simulink library "HEMERO"  (Simulink 3.00)
values from neighbouring files (symbols this model uses):
  K1 = 0.5    [ejh64.m]    (also in ejh65.m)
  K2 = 0.8    [ejh64.m]    (also in ejh65.m)
  x_camino = 0:0.01:10    [ejh64.m]    (also in ejh65.m)
  y_camino = x_camino.^2    [ejh64.m]    (also in ejh65.m)
undefined symbols (not defined in the file or in its folder): magnitude, nonlinear
libraries: simulink_extras x12, HEMERO x9, simulink3 x6, dspstat x4
(part 8 of 9)

== system HEMERO/Robots móviles/Control de robots móviles/Métodos basados en Teoría de Control/Seguimiento de trayectorias/Ejemplos/Ejemplo H.6.6/Seguimiento de trayectorias (Control lineal)/Control lineal/Cálculo de u1 ==
  e1 : Inport  Port=1  PortWidth=-1  SampleTime=-1  DataType=auto
      settings: SignalType=auto
  Gain : Gain  Gain=-K1  SaturateOnIntegerOverflow=on
  u1 : Outport  Port=1
  wires:
  e1/1 -> Gain/1
  Gain/1 -> u1/1

== system HEMERO/Robots móviles/Control de robots móviles/Métodos basados en Teoría de Control/Seguimiento de trayectorias/Ejemplos/Ejemplo H.6.6/Seguimiento de trayectorias (Control lineal)/Control lineal/Cálculo de u2  ==
  e2 : Inport  Port=1  PortWidth=-1  SampleTime=-1  DataType=auto
      settings: SignalType=auto
  e3 : Inport  Port=2  PortWidth=-1  SampleTime=-1  DataType=auto
      settings: SignalType=auto
  v_r : Inport  Port=3  PortWidth=-1  SampleTime=-1  DataType=auto
      settings: SignalType=auto
  Gain1 : Gain  Gain=-K2  SaturateOnIntegerOverflow=on
  Gain3 : Gain  Gain=-K3  SaturateOnIntegerOverflow=on
  Product1 : Product  Inputs=2  SaturateOnIntegerOverflow=on
  Sign : Signum
  Sum : Sum  Inputs=++  SaturateOnIntegerOverflow=on
  u2 : Outport  Port=1
  wires:
  Gain1/1 -> Product1/1
  Product1/1 -> Sum/1
  Sum/1 -> u2/1
  e3/1 -> Gain3/1
  Gain3/1 -> Sum/2
  e2/1 -> Gain1/1
  v_r/1 -> Sign/1
  Sign/1 -> Product1/2

== system HEMERO/Robots móviles/Control de robots móviles/Métodos basados en Teoría de Control/Seguimiento de trayectorias/Ejemplos/Ejemplo H.6.7/Seguimiento de trayectorias (Control lineal con escalado de velocidad)/Cambio de variable/Cálculo de e1 ==
  x_r : Inport  Port=1  PortWidth=-1  SampleTime=-1  DataType=auto
      settings: SignalType=auto
  x : Inport  Port=2  PortWidth=-1  SampleTime=-1  DataType=auto
      settings: SignalType=auto
  y_r : Inport  Port=3  PortWidth=-1  SampleTime=-1  DataType=auto
      settings: SignalType=auto
  y : Inport  Port=4  PortWidth=-1  SampleTime=-1  DataType=auto
      settings: SignalType=auto
  phi : Inport  Port=5  PortWidth=-1  SampleTime=-1  DataType=auto
      settings: SignalType=auto
  Product : Product  Inputs=2  SaturateOnIntegerOverflow=on
  Product1 : Product  Inputs=2  SaturateOnIntegerOverflow=on
  Sum : Sum  Inputs=-+  SaturateOnIntegerOverflow=on
  Sum1 : Sum  Inputs=+-  SaturateOnIntegerOverflow=on
  Sum2 : Sum  Inputs=++  SaturateOnIntegerOverflow=on
  Trigonometric Function : Trigonometry  Operator=sin  OutputSignalType=auto
  Trigonometric Function1 : Trigonometry  Operator=cos  OutputSignalType=auto
  e1 : Outport  Port=1
  wires:
  x_r/1 -> Sum/1
  x/1 -> Sum/2
  y_r/1 -> Sum1/1
  y/1 -> Sum1/2
  phi/1 -> Trigonometric Function/1, Trigonometric Function1/1
  Sum/1 -> Product/1
  Trigonometric Function/1 -> Product/2
  Sum1/1 -> Product1/1
  Trigonometric Function1/1 -> Product1/2
  Product/1 -> Sum2/1
  Product1/1 -> Sum2/2
  Sum2/1 -> e1/1

== system HEMERO/Robots móviles/Control de robots móviles/Métodos basados en Teoría de Control/Seguimiento de trayectorias/Ejemplos/Ejemplo H.6.7/Seguimiento de trayectorias (Control lineal con escalado de velocidad)/Cambio de variable/Cálculo de e2 ==
  x_r : Inport  Port=1  PortWidth=-1  SampleTime=-1  DataType=auto
      settings: SignalType=auto
  x : Inport  Port=2  PortWidth=-1  SampleTime=-1  DataType=auto
      settings: SignalType=auto
  y_r : Inport  Port=3  PortWidth=-1  SampleTime=-1  DataType=auto
      settings: SignalType=auto
  y : Inport  Port=4  PortWidth=-1  SampleTime=-1  DataType=auto
      settings: SignalType=auto
  phi : Inport  Port=5  PortWidth=-1  SampleTime=-1  DataType=auto
      settings: SignalType=auto
  Product : Product  Inputs=2  SaturateOnIntegerOverflow=on
  Product1 : Product  Inputs=2  SaturateOnIntegerOverflow=on
  Sum : Sum  Inputs=-+  SaturateOnIntegerOverflow=on
  Sum1 : Sum  Inputs=-+  SaturateOnIntegerOverflow=on
  Sum2 : Sum  Inputs=++  SaturateOnIntegerOverflow=on
  Trigonometric Function2 : Trigonometry  Operator=sin  OutputSignalType=auto
  Trigonometric Function3 : Trigonometry  Operator=cos  OutputSignalType=auto
  e2 : Outport  Port=1
  wires:
  x_r/1 -> Sum/1
  x/1 -> Sum/2
  y_r/1 -> Sum1/1
  y/1 -> Sum1/2
  phi/1 -> Trigonometric Function3/1, Trigonometric Function2/1
  Sum/1 -> Product/1
  Trigonometric Function3/1 -> Product/2
  Sum1/1 -> Product1/1
  Trigonometric Function2/1 -> Product1/2
  Product/1 -> Sum2/1
  Product1/1 -> Sum2/2
  Sum2/1 -> e2/1

== system HEMERO/Robots móviles/Control de robots móviles/Métodos basados en Teoría de Control/Seguimiento de trayectorias/Ejemplos/Ejemplo H.6.7/Seguimiento de trayectorias (Control lineal con escalado de velocidad)/Cambio de variable/Cálculo de e3 ==
  phi_r : Inport  Port=1  PortWidth=-1  SampleTime=-1  DataType=auto
      settings: SignalType=auto
  phi : Inport  Port=2  PortWidth=-1  SampleTime=-1  DataType=auto
      settings: SignalType=auto
  Subsystem2 : Subsystem
      mask Description: Pasa phi gorro al intervalo -180,180
  suma : Sum  Inputs=+-  SaturateOnIntegerOverflow=on
  e3 : Outport  Port=1
  wires:
  phi/1 -> suma/2
  phi_r/1 -> suma/1
  suma/1 -> Subsystem2/1(phi_gorro)
  Subsystem2/1(phi_go_mod) -> e3/1

== system HEMERO/Robots móviles/Control de robots móviles/Métodos basados en Teoría de Control/Seguimiento de trayectorias/Ejemplos/Ejemplo H.6.7/Seguimiento de trayectorias (Control lineal con escalado de velocidad)/Control lineal con escalado de velocidad/Cálculo de u1 ==
  e1 : Inport  Port=1  PortWidth=-1  SampleTime=-1  DataType=auto
      settings: SignalType=auto
  v_r : Inport  Port=2  PortWidth=-1  SampleTime=-1  DataType=auto
      settings: SignalType=auto
  w_r : Inport  Port=3  PortWidth=-1  SampleTime=-1  DataType=auto
      settings: SignalType=auto
  Constant : Constant  Value=b
  Fcn : Fcn  Expr=u^2
  Fcn1 : Fcn  Expr=u^2
  Fcn2 : Fcn  Expr=sqrt(u)
  Gain : Gain  Gain=-1  SaturateOnIntegerOverflow=on
  Gain1 : Gain  Gain=2*d  SaturateOnIntegerOverflow=on
  Product : Product  Inputs=2  SaturateOnIntegerOverflow=on
  Product1 : Product  Inputs=2  SaturateOnIntegerOverflow=on
  Sum : Sum  Inputs=++  SaturateOnIntegerOverflow=on
  u1 : Outport  Port=1
  K1 : Outport  Port=2
  wires:
  e1/1 -> Gain/1
  w_r/1 -> Fcn/1
  v_r/1 -> Fcn1/1
  Fcn1/1 -> Product/1
  Constant/1 -> Product/2
  Product/1 -> Sum/1
  Fcn/1 -> Sum/2
  Sum/1 -> Fcn2/1
  Gain/1 -> Product1/1
  Product1/1 -> u1/1
  Fcn2/1 -> Gain1/1
  Gain1/1 -> Product1/2, K1/1

== system HEMERO/Robots móviles/Control de robots móviles/Métodos basados en Teoría de Control/Seguimiento de trayectorias/Ejemplos/Ejemplo H.6.7/Seguimiento de trayectorias (Control lineal con escalado de velocidad)/Control lineal con escalado de velocidad/Cálculo de u2  ==
  note: K2
  e2 : Inport  Port=1  PortWidth=-1  SampleTime=-1  DataType=auto
      settings: SignalType=auto
  e3 : Inport  Port=2  PortWidth=-1  SampleTime=-1  DataType=auto
      settings: SignalType=auto
  v_r : Inport  Port=3  PortWidth=-1  SampleTime=-1  DataType=auto
      settings: SignalType=auto
  K3 : Inport  Port=4  PortWidth=-1  SampleTime=-1  DataType=auto
      settings: SignalType=auto
  Abs : Abs
  Gain1 : Gain  Gain=-1  SaturateOnIntegerOverflow=on
  Gain2 : Gain  Gain=b  SaturateOnIntegerOverflow=on
  Product : Product  Inputs=2  SaturateOnIntegerOverflow=on
  Product1 : Product  Inputs=2  SaturateOnIntegerOverflow=on
  Product3 : Product  Inputs=2  SaturateOnIntegerOverflow=on
  Sign : Signum
  Sum : Sum  Inputs=+-  SaturateOnIntegerOverflow=on
  u2 : Outport  Port=1
  wires:
  Sign/1 -> Product/2
  e2/1 -> Product/1
  Product/1 -> Gain1/1
  v_r/1 -> Sign/1, Abs/1
  Abs/1 -> Gain2/1
  Gain1/1 -> Product1/1
  Gain2/1 -> Product1/2
  Product1/1 -> Sum/1
  e3/1 -> Product3/1
  Sum/1 -> u2/1
  Product3/1 -> Sum/2
  K3/1 -> Product3/2

== system HEMERO/Robots móviles/Control de robots móviles/Métodos basados en Teoría de Control/Seguimiento de trayectorias/Ejemplos/Ejemplo H.6.8/Seguimiento de trayectorias (Control no lineal)/Cambio de variable/Cálculo de e1 ==
  x_r : Inport  Port=1  PortWidth=-1  SampleTime=-1  DataType=auto
      settings: SignalType=auto
  x : Inport  Port=2  PortWidth=-1  SampleTime=-1  DataType=auto
      settings: SignalType=auto
  y_r : Inport  Port=3  PortWidth=-1  SampleTime=-1  DataType=auto
      settings: SignalType=auto
  y : Inport  Port=4  PortWidth=-1  SampleTime=-1  DataType=auto
      settings: SignalType=auto
  phi : Inport  Port=5  PortWidth=-1  SampleTime=-1  DataType=auto
      settings: SignalType=auto
  Product : Product  Inputs=2  SaturateOnIntegerOverflow=on
  Product1 : Product  Inputs=2  SaturateOnIntegerOverflow=on
  Sum : Sum  Inputs=-+  SaturateOnIntegerOverflow=on
  Sum1 : Sum  Inputs=+-  SaturateOnIntegerOverflow=on
  Sum2 : Sum  Inputs=++  SaturateOnIntegerOverflow=on
  Trigonometric Function : Trigonometry  Operator=sin  OutputSignalType=auto
  Trigonometric Function1 : Trigonometry  Operator=cos  OutputSignalType=auto
  e1 : Outport  Port=1
  wires:
  x_r/1 -> Sum/1
  x/1 -> Sum/2
  y_r/1 -> Sum1/1
  y/1 -> Sum1/2
  phi/1 -> Trigonometric Function/1, Trigonometric Function1/1
  Sum/1 -> Product/1
  Trigonometric Function/1 -> Product/2
  Sum1/1 -> Product1/1
  Trigonometric Function1/1 -> Product1/2
  Product/1 -> Sum2/1
  Product1/1 -> Sum2/2
  Sum2/1 -> e1/1

== system HEMERO/Robots móviles/Control de robots móviles/Métodos basados en Teoría de Control/Seguimiento de trayectorias/Ejemplos/Ejemplo H.6.8/Seguimiento de trayectorias (Control no lineal)/Cambio de variable/Cálculo de e2 ==
  x_r : Inport  Port=1  PortWidth=-1  SampleTime=-1  DataType=auto
      settings: SignalType=auto
  x : Inport  Port=2  PortWidth=-1  SampleTime=-1  DataType=auto
      settings: SignalType=auto
  y_r : Inport  Port=3  PortWidth=-1  SampleTime=-1  DataType=auto
      settings: SignalType=auto
  y : Inport  Port=4  PortWidth=-1  SampleTime=-1  DataType=auto
      settings: SignalType=auto
  phi : Inport  Port=5  PortWidth=-1  SampleTime=-1  DataType=auto
      settings: SignalType=auto
  Product : Product  Inputs=2  SaturateOnIntegerOverflow=on
  Product1 : Product  Inputs=2  SaturateOnIntegerOverflow=on
  Sum : Sum  Inputs=-+  SaturateOnIntegerOverflow=on
  Sum1 : Sum  Inputs=-+  SaturateOnIntegerOverflow=on
  Sum2 : Sum  Inputs=++  SaturateOnIntegerOverflow=on
  Trigonometric Function2 : Trigonometry  Operator=sin  OutputSignalType=auto
  Trigonometric Function3 : Trigonometry  Operator=cos  OutputSignalType=auto
  e2 : Outport  Port=1
  wires:
  x_r/1 -> Sum/1
  x/1 -> Sum/2
  y_r/1 -> Sum1/1
  y/1 -> Sum1/2
  phi/1 -> Trigonometric Function3/1, Trigonometric Function2/1
  Sum/1 -> Product/1
  Trigonometric Function3/1 -> Product/2
  Sum1/1 -> Product1/1
  Trigonometric Function2/1 -> Product1/2
  Product/1 -> Sum2/1
  Product1/1 -> Sum2/2
  Sum2/1 -> e2/1

== system HEMERO/Robots móviles/Control de robots móviles/Métodos basados en Teoría de Control/Seguimiento de trayectorias/Ejemplos/Ejemplo H.6.8/Seguimiento de trayectorias (Control no lineal)/Cambio de variable/Cálculo de e3 ==
  phi_r : Inport  Port=1  PortWidth=-1  SampleTime=-1  DataType=auto
      settings: SignalType=auto
  phi : Inport  Port=2  PortWidth=-1  SampleTime=-1  DataType=auto
      settings: SignalType=auto
  Subsystem2 : Subsystem
      mask Description: Pasa phi gorro al intervalo -180,180
  suma : Sum  Inputs=+-  SaturateOnIntegerOverflow=on
  e3 : Outport  Port=1
  wires:
  phi/1 -> suma/2
  phi_r/1 -> suma/1
  suma/1 -> Subsystem2/1(phi_gorro)
  Subsystem2/1(phi_go_mod) -> e3/1

== system HEMERO/Robots móviles/Control de robots móviles/Métodos basados en Teoría de Control/Seguimiento de trayectorias/Ejemplos/Ejemplo H.6.8/Seguimiento de trayectorias (Control no lineal)/Control no lineal/Cálculo de u1 ==
  e1 : Inport  Port=1  PortWidth=-1  SampleTime=-1  DataType=auto
      settings: SignalType=auto
  K1 : Inport  Port=2  PortWidth=-1  SampleTime=-1  DataType=auto
      settings: SignalType=auto
  Gain : Gain  Gain=-1  SaturateOnIntegerOverflow=on
  Product : Product  Inputs=2  SaturateOnIntegerOverflow=on
  u1 : Outport  Port=1
  wires:
  e1/1 -> Product/1
  Product/1 -> u1/1
  K1/1 -> Gain/1
  Gain/1 -> Product/2

== system HEMERO/Robots móviles/Control de robots móviles/Métodos basados en Teoría de Control/Seguimiento de trayectorias/Ejemplos/Ejemplo H.6.8/Seguimiento de trayectorias (Control no lineal)/Control no lineal/Cálculo de u2  ==
  e2 : Inport  Port=1  PortWidth=-1  SampleTime=-1  DataType=auto
      settings: SignalType=auto
  e3 : Inport  Port=2  PortWidth=-1  SampleTime=-1  DataType=auto
      settings: SignalType=auto
  v_r : Inport  Port=3  PortWidth=-1  SampleTime=-1  DataType=auto
      settings: SignalType=auto
  K3 : Inport  Port=4  PortWidth=-1  SampleTime=-1  DataType=auto
      settings: SignalType=auto
  Gain1 : Gain  Gain=-K2  SaturateOnIntegerOverflow=on
  Gain2 : Gain  Gain=-1  SaturateOnIntegerOverflow=on
  MATLAB Fcn : MATLABFcn  MATLABFcn=nonlinear(u)  OutputWidth=-1  OutputSignalType=auto
  Product1 : Product  Inputs=3  SaturateOnIntegerOverflow=on
  Product2 : Product  Inputs=2  SaturateOnIntegerOverflow=on
  Sum : Sum  Inputs=++  SaturateOnIntegerOverflow=on
  u2 : Outport  Port=1
  wires:
  MATLAB Fcn/1 -> Product1/3
  Gain1/1 -> Product1/1
  Product1/1 -> Sum/1
  Sum/1 -> u2/1
  e2/1 -> Gain1/1
  K3/1 -> Gain2/1
  Gain2/1 -> Product2/2
  Product2/1 -> Sum/2
  v_r/1 -> Product1/2
  e3/1 -> MATLAB Fcn/1, Product2/1

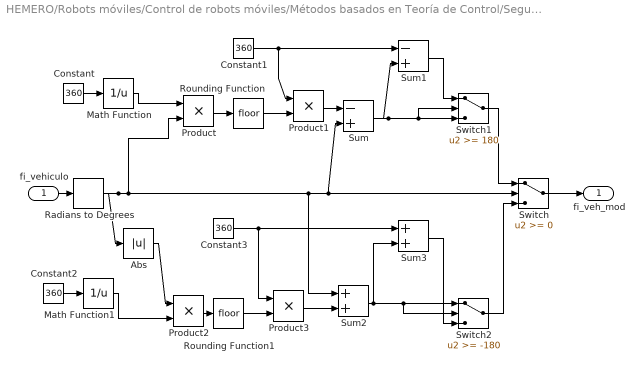
== system HEMERO/Robots móviles/Control de robots móviles/Métodos basados en Teoría de Control/Seguimiento de caminos/Ejemplos/Ejemplo H.6.4/Seguimiento de caminos (control lineal)/Cálculo de parámetros/Cálculo de phi gorro/Subsystem ==
  fi_vehiculo : Inport  Port=1  PortWidth=-1  SampleTime=-1  DataType=auto
      settings: SignalType=auto
  Abs : Abs
  Constant{,1..3} (4 alike) : Constant  Value=360
  Math Function : Math  Operator=reciprocal  OutputSignalType=auto
  Math Function1 : Math  Operator=reciprocal  OutputSignalType=auto
  Product{,1..3} (4 alike) : Product  Inputs=2  SaturateOnIntegerOverflow=on
  Radians to Degrees : simulink_extras/Transformations/Radians to Degrees
  Rounding Function : Rounding  Operator=floor
  Rounding Function1 : Rounding  Operator=floor
  Sum : Sum  Inputs=-+  SaturateOnIntegerOverflow=on
  Sum1 : Sum  Inputs=-+  SaturateOnIntegerOverflow=on
  Sum2 : Sum  Inputs=++  SaturateOnIntegerOverflow=on
  Sum3 : Sum  Inputs=++  SaturateOnIntegerOverflow=on
  Switch : Switch  Threshold=0
  Switch1 : Switch  Threshold=180
  Switch2 : Switch  Threshold=-180
  fi_veh_mod : Outport  Port=1
  wires:
  Radians to Degrees/1 -> Abs/1, Sum2/1, Sum/2, Switch/2, Product/2
  fi_vehiculo/1 -> Radians to Degrees/1
  Abs/1 -> Product2/1
  Sum2/1 -> Switch2/2, Switch2/1, Sum3/2
  Sum3/1 -> Switch2/3
  Product2/1 -> Rounding Function1/1
  Math Function1/1 -> Product2/2
  Constant2/1 -> Math Function1/1
  Product3/1 -> Sum2/2
  Rounding Function1/1 -> Product3/2
  Switch2/1 -> Switch/3
  Constant3/1 -> Sum3/1, Product3/1
  Sum1/1 -> Switch1/1
  Sum/1 -> Switch1/2, Switch1/3, Sum1/2
  Constant1/1 -> Sum1/1, Product1/1
  Product1/1 -> Sum/1
  Rounding Function/1 -> Product1/2
  Product/1 -> Rounding Function/1
  Constant/1 -> Math Function/1
  Math Function/1 -> Product/1
  Switch1/1 -> Switch/1
  Switch/1 -> fi_veh_mod/1

== system HEMERO/Robots móviles/Control de robots móviles/Métodos basados en Teoría de Control/Seguimiento de caminos/Ejemplos/Ejemplo H.6.4/Seguimiento de caminos (control lineal)/Cálculo de parámetros/Cálculo de phi gorro/Subsystem1 ==
  indice : Inport  Port=1  PortWidth=-1  SampleTime=-1  DataType=auto
      settings: SignalType=auto
  Constant : Constant  Value=90
  Constant1 : Constant  Value=360
  Look-Up Table : Lookup  InputValues=1:length(der_x)  OutputValues=der_x(1:length(der_x))
  Look-Up Table1 : Lookup  InputValues=1:length(der_y)  OutputValues=der_y(1:length(der_y))
  Radians to Degrees : simulink_extras/Transformations/Radians to Degrees
  Sum : Sum  Inputs=+-  SaturateOnIntegerOverflow=on
  Sum1 : Sum  Inputs=++  SaturateOnIntegerOverflow=on
  Switch : Switch  Threshold=-180
  Trigonometric Function : Trigonometry  Operator=atan2  OutputSignalType=auto
  fi_camino : Outport  Port=1
  wires:
  indice/1 -> Look-Up Table/1, Look-Up Table1/1
  Switch/1 -> fi_camino/1
  Sum1/1 -> Switch/3
  Sum/1 -> Switch/2, Sum1/1, Switch/1
  Constant1/1 -> Sum1/2
  Constant/1 -> Sum/2
  Radians to Degrees/1 -> Sum/1
  Trigonometric Function/1 -> Radians to Degrees/1
  Look-Up Table/1 -> Trigonometric Function/2
  Look-Up Table1/1 -> Trigonometric Function/1

== system HEMERO/Robots móviles/Control de robots móviles/Métodos basados en Teoría de Control/Seguimiento de caminos/Ejemplos/Ejemplo H.6.4/Seguimiento de caminos (control lineal)/Cálculo de parámetros/Cálculo de phi gorro/Subsystem2 ==
  fi_gorro : Inport  Port=1  PortWidth=-1  SampleTime=-1  DataType=auto
      settings: SignalType=auto
  Constant1 : Constant  Value=360
  Constant2 : Constant  Value=360
  Sum1 : Sum  Inputs=-+  SaturateOnIntegerOverflow=on
  Sum2 : Sum  Inputs=++  SaturateOnIntegerOverflow=on
  Switch : Switch  Threshold=180
  Switch1 : Switch  Threshold=0
  Switch2 : Switch  Threshold=-180
  fi_go_mo : Outport  Port=1
  wires:
  Constant2/1 -> Sum2/2
  fi_gorro/1 -> Sum2/1, Switch2/2, Switch2/1, Switch/2, Switch/3, Switch1/2, Sum1/2
  Sum2/1 -> Switch2/3
  Sum1/1 -> Switch/1
  Constant1/1 -> Sum1/1
  Switch2/1 -> Switch1/3
  Switch/1 -> Switch1/1
  Switch1/1 -> fi_go_mo/1

== system HEMERO/Robots móviles/Control de robots móviles/Métodos basados en Teoría de Control/Seguimiento de caminos/Ejemplos/Ejemplo H.6.4/Seguimiento de caminos (control lineal)/Cálculo de parámetros/Subsystem/Parametros de Curvatura ==
  x_1 : Inport  Port=1  PortWidth=-1  SampleTime=-1  DataType=auto
      settings: SignalType=auto
  x_2 : Inport  Port=2  PortWidth=-1  SampleTime=-1  DataType=auto
      settings: SignalType=auto
  x_3 : Inport  Port=3  PortWidth=-1  SampleTime=-1  DataType=auto
      settings: SignalType=auto
  y_1 : Inport  Port=4  PortWidth=-1  SampleTime=-1  DataType=auto
      settings: SignalType=auto
  y_2 : Inport  Port=5  PortWidth=-1  SampleTime=-1  DataType=auto
      settings: SignalType=auto
  y_3 : Inport  Port=6  PortWidth=-1  SampleTime=-1  DataType=auto
      settings: SignalType=auto
  Radio de  Curvatura : Subsystem
  coordenada x c. curvatura : Subsystem
  coordenada y c. curvatura : Subsystem
  x_g : Outport  Port=1  InitialOutput=0
  y_g : Outport  Port=2  InitialOutput=0
  R_c : Outport  Port=3  InitialOutput=0
  wires:
  y_3/1 -> coordenada x c. curvatura/6(y_3), coordenada y c. curvatura/6(y_3)
  y_2/1 -> coordenada y c. curvatura/5(y_2), coordenada x c. curvatura/5(y_2)
  y_1/1 -> Radio de  Curvatura/4(y_1), coordenada x c. curvatura/4(y_1), coordenada y c. curvatura/4(y_1)
  x_3/1 -> coordenada y c. curvatura/3(x_3), coordenada x c. curvatura/3(x_3)
  x_2/1 -> coordenada y c. curvatura/2(x_2), coordenada x c. curvatura/2(x_2)
  x_1/1 -> Radio de  Curvatura/2(x_1), coordenada y c. curvatura/1(x_1), coordenada x c. curvatura/1(x_1)
  coordenada x c. curvatura/1(x_g) -> Radio de  Curvatura/1(x_g), x_g/1
  coordenada y c. curvatura/1(y_g) -> Radio de  Curvatura/3(y_g), y_g/1
  Radio de  Curvatura/1(R_c) -> R_c/1

== system HEMERO/Robots móviles/Control de robots móviles/Métodos basados en Teoría de Control/Seguimiento de caminos/Ejemplos/Ejemplo H.6.4/Seguimiento de caminos (control lineal)/Cálculo de parámetros/Subsystem/Subsystem ==
  x : Inport  Port=1  PortWidth=-1  SampleTime=-1  DataType=auto
      settings: SignalType=auto
  y : Inport  Port=2  PortWidth=-1  SampleTime=-1  DataType=auto
      settings: SignalType=auto
  x_g : Inport  Port=3  PortWidth=-1  SampleTime=-1  DataType=auto
      settings: SignalType=auto
  y_g : Inport  Port=4  PortWidth=-1  SampleTime=-1  DataType=auto
      settings: SignalType=auto
  Math Function2 : Math  Operator=sqrt  OutputSignalType=auto
  Math Function3 : Math  Operator=square  OutputSignalType=auto
  Math Function4 : Math  Operator=square  OutputSignalType=auto
  Sum : Sum  Inputs=+-  SaturateOnIntegerOverflow=on
  Sum1 : Sum  Inputs=+-  SaturateOnIntegerOverflow=on
  Sum2 : Sum  Inputs=++  SaturateOnIntegerOverflow=on
  dist : Outport  Port=1  InitialOutput=0
  wires:
  Sum2/1 -> Math Function2/1
  Math Function4/1 -> Sum2/2
  Sum1/1 -> Math Function4/1
  Math Function3/1 -> Sum2/1
  Sum/1 -> Math Function3/1
  y/1 -> Sum1/1
  x_g/1 -> Sum/2
  x/1 -> Sum/1
  y_g/1 -> Sum1/2
  Math Function2/1 -> dist/1

== system HEMERO/Robots móviles/Control de robots móviles/Métodos basados en Teoría de Control/Seguimiento de caminos/Ejemplos/Ejemplo H.6.4/Seguimiento de caminos (control lineal)/Cálculo de parámetros/Subsystem/distancia mínima1 ==
  x_camino : Inport  Port=1  PortWidth=-1  SampleTime=-1  DataType=auto
      settings: SignalType=auto
  y_camino : Inport  Port=2  PortWidth=-1  SampleTime=-1  DataType=auto
      settings: SignalType=auto
  x_vehiculo : Inport  Port=3  PortWidth=-1  SampleTime=-1  DataType=auto
      settings: SignalType=auto
  y_vehiculo : Inport  Port=4  PortWidth=-1  SampleTime=-1  DataType=auto
      settings: SignalType=auto
  Math Function2 : Math  Operator=sqrt  OutputSignalType=auto
  Math Function3 : Math  Operator=square  OutputSignalType=auto
  Math Function4 : Math  Operator=square  OutputSignalType=auto
  Minimum : dspstat/Minimum
  Sum : Sum  Inputs=+-  SaturateOnIntegerOverflow=on
  Sum1 : Sum  Inputs=+-  SaturateOnIntegerOverflow=on
  Sum2 : Sum  Inputs=++  SaturateOnIntegerOverflow=on
  d_min : Outport  Port=1  InitialOutput=0
  indice : Outport  Port=2  InitialOutput=0
  wires:
  Minimum/2 -> indice/1
  Minimum/1 -> d_min/1
  Math Function2/1 -> Minimum/1
  Sum2/1 -> Math Function2/1
  Math Function4/1 -> Sum2/2
  Sum1/1 -> Math Function4/1
  Math Function3/1 -> Sum2/1
  Sum/1 -> Math Function3/1
  y_vehiculo/1 -> Sum1/2
  y_camino/1 -> Sum1/1
  x_vehiculo/1 -> Sum/2
  x_camino/1 -> Sum/1

== system HEMERO/Robots móviles/Control de robots móviles/Métodos basados en Teoría de Control/Seguimiento de caminos/Ejemplos/Ejemplo H.6.4/Seguimiento de caminos (control lineal)/Cálculo de parámetros/Subsystem/tres_puntos ==
  indice : Inport  Port=1  PortWidth=-1  SampleTime=-1  DataType=auto
      settings: SignalType=auto
  Constant : Constant  Value=1
  Constant1 : Constant  Value=2
  Look-Up Table : Lookup  InputValues=1:length(x_camino)  OutputValues=x_camino(1:length(x_camino))
  Look-Up Table1 : Lookup  InputValues=1:length(y_camino)  OutputValues=y_camino(1:length(y_camino))
  Look-Up Table2 : Lookup  InputValues=1:length(x_camino)  OutputValues=x_camino(1:length(x_camino))
  Look-Up Table3 : Lookup  InputValues=1:length(y_camino)  OutputValues=y_camino(1:length(y_camino))
  Look-Up Table4 : Lookup  InputValues=1:length(x_camino)  OutputValues=x_camino(1:length(x_camino))
  Look-Up Table5 : Lookup  InputValues=1:length(y_camino)  OutputValues=y_camino(1:length(y_camino))
  Sum : Sum  Inputs=++  SaturateOnIntegerOverflow=on
  Sum1 : Sum  Inputs=++  SaturateOnIntegerOverflow=on
  x_1 : Outport  Port=1
  x_2 : Outport  Port=2
  x_3 : Outport  Port=3
  y_1 : Outport  Port=4
  y_2 : Outport  Port=5
  y_3 : Outport  Port=6
  wires:
  Sum1/1 -> Look-Up Table5/1, Look-Up Table4/1
  Look-Up Table4/1 -> x_3/1
  Look-Up Table5/1 -> y_3/1
  Constant1/1 -> Sum1/2
  Look-Up Table1/1 -> y_1/1
  Sum/1 -> Look-Up Table3/1, Look-Up Table2/1
  Look-Up Table3/1 -> y_2/1
  Look-Up Table2/1 -> x_2/1
  Constant/1 -> Sum/2
  indice/1 -> Sum1/1, Sum/1, Look-Up Table1/1, Look-Up Table/1
  Look-Up Table/1 -> x_1/1

== system HEMERO/Robots móviles/Control de robots móviles/Métodos basados en Teoría de Control/Seguimiento de caminos/Ejemplos/Ejemplo H.6.5/Seguimiento de caminos (control no lineal)/Cálculo de parámetros/Cálculo de phi gorro/Subsystem ==
  fi_vehiculo : Inport  Port=1  PortWidth=-1  SampleTime=-1  DataType=auto
      settings: SignalType=auto
  Abs : Abs
  Constant{,1..3} (4 alike) : Constant  Value=360
  Math Function : Math  Operator=reciprocal  OutputSignalType=auto
  Math Function1 : Math  Operator=reciprocal  OutputSignalType=auto
  Product{,1..3} (4 alike) : Product  Inputs=2  SaturateOnIntegerOverflow=on
  Radians to Degrees : simulink_extras/Transformations/Radians to Degrees
  Rounding Function : Rounding  Operator=floor
  Rounding Function1 : Rounding  Operator=floor
  Sum : Sum  Inputs=-+  SaturateOnIntegerOverflow=on
  Sum1 : Sum  Inputs=-+  SaturateOnIntegerOverflow=on
  Sum2 : Sum  Inputs=++  SaturateOnIntegerOverflow=on
  Sum3 : Sum  Inputs=++  SaturateOnIntegerOverflow=on
  Switch : Switch  Threshold=0
  Switch1 : Switch  Threshold=180
  Switch2 : Switch  Threshold=-180
  fi_veh_mod : Outport  Port=1
  wires:
  Radians to Degrees/1 -> Abs/1, Sum2/1, Sum/2, Switch/2, Product/2
  fi_vehiculo/1 -> Radians to Degrees/1
  Abs/1 -> Product2/1
  Sum2/1 -> Switch2/2, Switch2/1, Sum3/2
  Sum3/1 -> Switch2/3
  Product2/1 -> Rounding Function1/1
  Math Function1/1 -> Product2/2
  Constant2/1 -> Math Function1/1
  Product3/1 -> Sum2/2
  Rounding Function1/1 -> Product3/2
  Switch2/1 -> Switch/3
  Constant3/1 -> Sum3/1, Product3/1
  Sum1/1 -> Switch1/1
  Sum/1 -> Switch1/2, Switch1/3, Sum1/2
  Constant1/1 -> Sum1/1, Product1/1
  Product1/1 -> Sum/1
  Rounding Function/1 -> Product1/2
  Product/1 -> Rounding Function/1
  Constant/1 -> Math Function/1
  Math Function/1 -> Product/1
  Switch1/1 -> Switch/1
  Switch/1 -> fi_veh_mod/1

== system HEMERO/Robots móviles/Control de robots móviles/Métodos basados en Teoría de Control/Seguimiento de caminos/Ejemplos/Ejemplo H.6.5/Seguimiento de caminos (control no lineal)/Cálculo de parámetros/Cálculo de phi gorro/Subsystem1 ==
  indice : Inport  Port=1  PortWidth=-1  SampleTime=-1  DataType=auto
      settings: SignalType=auto
  Constant : Constant  Value=90
  Constant1 : Constant  Value=360
  Look-Up Table : Lookup  InputValues=1:length(der_x)  OutputValues=der_x(1:length(der_x))
  Look-Up Table1 : Lookup  InputValues=1:length(der_y)  OutputValues=der_y(1:length(der_y))
  Radians to Degrees : simulink_extras/Transformations/Radians to Degrees
  Sum : Sum  Inputs=+-  SaturateOnIntegerOverflow=on
  Sum1 : Sum  Inputs=++  SaturateOnIntegerOverflow=on
  Switch : Switch  Threshold=-180
  Trigonometric Function : Trigonometry  Operator=atan2  OutputSignalType=auto
  fi_camino : Outport  Port=1
  wires:
  indice/1 -> Look-Up Table/1, Look-Up Table1/1
  Switch/1 -> fi_camino/1
  Sum1/1 -> Switch/3
  Sum/1 -> Switch/2, Sum1/1, Switch/1
  Constant1/1 -> Sum1/2
  Constant/1 -> Sum/2
  Radians to Degrees/1 -> Sum/1
  Trigonometric Function/1 -> Radians to Degrees/1
  Look-Up Table/1 -> Trigonometric Function/2
  Look-Up Table1/1 -> Trigonometric Function/1

== system HEMERO/Robots móviles/Control de robots móviles/Métodos basados en Teoría de Control/Seguimiento de caminos/Ejemplos/Ejemplo H.6.5/Seguimiento de caminos (control no lineal)/Cálculo de parámetros/Cálculo de phi gorro/Subsystem2 ==
  fi_gorro : Inport  Port=1  PortWidth=-1  SampleTime=-1  DataType=auto
      settings: SignalType=auto
  Constant1 : Constant  Value=360
  Constant2 : Constant  Value=360
  Sum1 : Sum  Inputs=-+  SaturateOnIntegerOverflow=on
  Sum2 : Sum  Inputs=++  SaturateOnIntegerOverflow=on
  Switch : Switch  Threshold=180
  Switch1 : Switch  Threshold=0
  Switch2 : Switch  Threshold=-180
  fi_go_mo : Outport  Port=1
  wires:
  Constant2/1 -> Sum2/2
  fi_gorro/1 -> Sum2/1, Switch2/2, Switch2/1, Switch/2, Switch/3, Switch1/2, Sum1/2
  Sum2/1 -> Switch2/3
  Sum1/1 -> Switch/1
  Constant1/1 -> Sum1/1
  Switch2/1 -> Switch1/3
  Switch/1 -> Switch1/1
  Switch1/1 -> fi_go_mo/1

== system HEMERO/Robots móviles/Control de robots móviles/Métodos basados en Teoría de Control/Seguimiento de caminos/Ejemplos/Ejemplo H.6.5/Seguimiento de caminos (control no lineal)/Cálculo de parámetros/Subsystem/Parametros de Curvatura ==
  x_1 : Inport  Port=1  PortWidth=-1  SampleTime=-1  DataType=auto
      settings: SignalType=auto
  x_2 : Inport  Port=2  PortWidth=-1  SampleTime=-1  DataType=auto
      settings: SignalType=auto
  x_3 : Inport  Port=3  PortWidth=-1  SampleTime=-1  DataType=auto
      settings: SignalType=auto
  y_1 : Inport  Port=4  PortWidth=-1  SampleTime=-1  DataType=auto
      settings: SignalType=auto
  y_2 : Inport  Port=5  PortWidth=-1  SampleTime=-1  DataType=auto
      settings: SignalType=auto
  y_3 : Inport  Port=6  PortWidth=-1  SampleTime=-1  DataType=auto
      settings: SignalType=auto
  Radio de  Curvatura : Subsystem
  coordenada x c. curvatura : Subsystem
  coordenada y c. curvatura : Subsystem
  x_g : Outport  Port=1  InitialOutput=0
  y_g : Outport  Port=2  InitialOutput=0
  R_c : Outport  Port=3  InitialOutput=0
  wires:
  y_3/1 -> coordenada x c. curvatura/6(y_3), coordenada y c. curvatura/6(y_3)
  y_2/1 -> coordenada y c. curvatura/5(y_2), coordenada x c. curvatura/5(y_2)
  y_1/1 -> Radio de  Curvatura/4(y_1), coordenada x c. curvatura/4(y_1), coordenada y c. curvatura/4(y_1)
  x_3/1 -> coordenada y c. curvatura/3(x_3), coordenada x c. curvatura/3(x_3)
  x_2/1 -> coordenada y c. curvatura/2(x_2), coordenada x c. curvatura/2(x_2)
  x_1/1 -> Radio de  Curvatura/2(x_1), coordenada y c. curvatura/1(x_1), coordenada x c. curvatura/1(x_1)
  coordenada x c. curvatura/1(x_g) -> Radio de  Curvatura/1(x_g), x_g/1
  coordenada y c. curvatura/1(y_g) -> Radio de  Curvatura/3(y_g), y_g/1
  Radio de  Curvatura/1(R_c) -> R_c/1

== system HEMERO/Robots móviles/Control de robots móviles/Métodos basados en Teoría de Control/Seguimiento de caminos/Ejemplos/Ejemplo H.6.5/Seguimiento de caminos (control no lineal)/Cálculo de parámetros/Subsystem/Subsystem ==
  x : Inport  Port=1  PortWidth=-1  SampleTime=-1  DataType=auto
      settings: SignalType=auto
  y : Inport  Port=2  PortWidth=-1  SampleTime=-1  DataType=auto
      settings: SignalType=auto
  x_g : Inport  Port=3  PortWidth=-1  SampleTime=-1  DataType=auto
      settings: SignalType=auto
  y_g : Inport  Port=4  PortWidth=-1  SampleTime=-1  DataType=auto
      settings: SignalType=auto
  Math Function2 : Math  Operator=sqrt  OutputSignalType=auto
  Math Function3 : Math  Operator=square  OutputSignalType=auto
  Math Function4 : Math  Operator=square  OutputSignalType=auto
  Sum : Sum  Inputs=+-  SaturateOnIntegerOverflow=on
  Sum1 : Sum  Inputs=+-  SaturateOnIntegerOverflow=on
  Sum2 : Sum  Inputs=++  SaturateOnIntegerOverflow=on
  dist : Outport  Port=1  InitialOutput=0
  wires:
  Sum2/1 -> Math Function2/1
  Math Function4/1 -> Sum2/2
  Sum1/1 -> Math Function4/1
  Math Function3/1 -> Sum2/1
  Sum/1 -> Math Function3/1
  y/1 -> Sum1/1
  x_g/1 -> Sum/2
  x/1 -> Sum/1
  y_g/1 -> Sum1/2
  Math Function2/1 -> dist/1

== system HEMERO/Robots móviles/Control de robots móviles/Métodos basados en Teoría de Control/Seguimiento de caminos/Ejemplos/Ejemplo H.6.5/Seguimiento de caminos (control no lineal)/Cálculo de parámetros/Subsystem/distancia mínima1 ==
  x_camino : Inport  Port=1  PortWidth=-1  SampleTime=-1  DataType=auto
      settings: SignalType=auto
  y_camino : Inport  Port=2  PortWidth=-1  SampleTime=-1  DataType=auto
      settings: SignalType=auto
  x_vehiculo : Inport  Port=3  PortWidth=-1  SampleTime=-1  DataType=auto
      settings: SignalType=auto
  y_vehiculo : Inport  Port=4  PortWidth=-1  SampleTime=-1  DataType=auto
      settings: SignalType=auto
  Math Function2 : Math  Operator=sqrt  OutputSignalType=auto
  Math Function3 : Math  Operator=square  OutputSignalType=auto
  Math Function4 : Math  Operator=square  OutputSignalType=auto
  Minimum : dspstat/Minimum
  Sum : Sum  Inputs=+-  SaturateOnIntegerOverflow=on
  Sum1 : Sum  Inputs=+-  SaturateOnIntegerOverflow=on
  Sum2 : Sum  Inputs=++  SaturateOnIntegerOverflow=on
  d_min : Outport  Port=1  InitialOutput=0
  indice : Outport  Port=2  InitialOutput=0
  wires:
  Minimum/2 -> indice/1
  Minimum/1 -> d_min/1
  Math Function2/1 -> Minimum/1
  Sum2/1 -> Math Function2/1
  Math Function4/1 -> Sum2/2
  Sum1/1 -> Math Function4/1
  Math Function3/1 -> Sum2/1
  Sum/1 -> Math Function3/1
  y_vehiculo/1 -> Sum1/2
  y_camino/1 -> Sum1/1
  x_vehiculo/1 -> Sum/2
  x_camino/1 -> Sum/1

== system HEMERO/Robots móviles/Control de robots móviles/Métodos basados en Teoría de Control/Seguimiento de caminos/Ejemplos/Ejemplo H.6.5/Seguimiento de caminos (control no lineal)/Cálculo de parámetros/Subsystem/tres_puntos ==
  indice : Inport  Port=1  PortWidth=-1  SampleTime=-1  DataType=auto
      settings: SignalType=auto
  Constant : Constant  Value=1
  Constant1 : Constant  Value=2
  Look-Up Table : Lookup  InputValues=1:length(x_camino)  OutputValues=x_camino(1:length(x_camino))
  Look-Up Table1 : Lookup  InputValues=1:length(y_camino)  OutputValues=y_camino(1:length(y_camino))
  Look-Up Table2 : Lookup  InputValues=1:length(x_camino)  OutputValues=x_camino(1:length(x_camino))
  Look-Up Table3 : Lookup  InputValues=1:length(y_camino)  OutputValues=y_camino(1:length(y_camino))
  Look-Up Table4 : Lookup  InputValues=1:length(x_camino)  OutputValues=x_camino(1:length(x_camino))
  Look-Up Table5 : Lookup  InputValues=1:length(y_camino)  OutputValues=y_camino(1:length(y_camino))
  Sum : Sum  Inputs=++  SaturateOnIntegerOverflow=on
  Sum1 : Sum  Inputs=++  SaturateOnIntegerOverflow=on
  x_1 : Outport  Port=1
  x_2 : Outport  Port=2
  x_3 : Outport  Port=3
  y_1 : Outport  Port=4
  y_2 : Outport  Port=5
  y_3 : Outport  Port=6
  wires:
  Sum1/1 -> Look-Up Table5/1, Look-Up Table4/1
  Look-Up Table4/1 -> x_3/1
  Look-Up Table5/1 -> y_3/1
  Constant1/1 -> Sum1/2
  Look-Up Table1/1 -> y_1/1
  Sum/1 -> Look-Up Table3/1, Look-Up Table2/1
  Look-Up Table3/1 -> y_2/1
  Look-Up Table2/1 -> x_2/1
  Constant/1 -> Sum/2
  indice/1 -> Sum1/1, Sum/1, Look-Up Table1/1, Look-Up Table/1
  Look-Up Table/1 -> x_1/1

== system HEMERO/Robots móviles/Control de robots móviles/Métodos basados en Teoría de Control/Seguimiento de caminos/Seguimiento de caminos (control lineal)/Cálculo de parámetros/Subsystem/Parametros de Curvatura/coordenada x c. curvatura/bloque_1 ==
  x1 : Inport  Port=1  PortWidth=-1  SampleTime=-1  DataType=auto
      settings: SignalType=auto
  x2 : Inport  Port=2  PortWidth=-1  SampleTime=-1  DataType=auto
      settings: SignalType=auto
  y1 : Inport  Port=3  PortWidth=-1  SampleTime=-1  DataType=auto
      settings: SignalType=auto
  y2 : Inport  Port=4  PortWidth=-1  SampleTime=-1  DataType=auto
      settings: SignalType=auto
  Gain : Gain  Gain=0.5  SaturateOnIntegerOverflow=on
  Math Function{,1..3} (4 alike) : Math  Operator=square  OutputSignalType=auto
  Sum : Sum  Inputs=-+  SaturateOnIntegerOverflow=on
  Sum1 : Sum  Inputs=-+  SaturateOnIntegerOverflow=on
  Sum2 : Sum  Inputs=-+-+  SaturateOnIntegerOverflow=on
  alfa_1 : Outport  Port=1  InitialOutput=0
  beta_1 : Outport  Port=2  InitialOutput=0
  c_1 : Outport  Port=3  InitialOutput=0
  wires:
  Gain/1 -> c_1/1
  Sum2/1 -> Gain/1
  Math Function3/1 -> Sum2/4
  Math Function2/1 -> Sum2/3
  Math Function1/1 -> Sum2/2
  Math Function/1 -> Sum2/1
  y2/1 -> Math Function3/1, Sum1/2
  y1/1 -> Math Function2/1, Sum1/1
  x2/1 -> Math Function1/1, Sum/2
  x1/1 -> Math Function/1, Sum/1
  Sum1/1 -> beta_1/1
  Sum/1 -> alfa_1/1

== system HEMERO/Robots móviles/Control de robots móviles/Métodos basados en Teoría de Control/Seguimiento de caminos/Seguimiento de caminos (control lineal)/Cálculo de parámetros/Subsystem/Parametros de Curvatura/coordenada x c. curvatura/bloque_2 ==
  x2 : Inport  Port=1  PortWidth=-1  SampleTime=-1  DataType=auto
      settings: SignalType=auto
  x3 : Inport  Port=2  PortWidth=-1  SampleTime=-1  DataType=auto
      settings: SignalType=auto
  y2 : Inport  Port=3  PortWidth=-1  SampleTime=-1  DataType=auto
      settings: SignalType=auto
  y3 : Inport  Port=4  PortWidth=-1  SampleTime=-1  DataType=auto
      settings: SignalType=auto
  Gain : Gain  Gain=0.5  SaturateOnIntegerOverflow=on
  Math Function{,1..3} (4 alike) : Math  Operator=square  OutputSignalType=auto
  Sum : Sum  Inputs=-+  SaturateOnIntegerOverflow=on
  Sum1 : Sum  Inputs=-+  SaturateOnIntegerOverflow=on
  Sum2 : Sum  Inputs=-+-+  SaturateOnIntegerOverflow=on
  alfa_2 : Outport  Port=1  InitialOutput=0
  beta_2 : Outport  Port=2  InitialOutput=0
  c_2 : Outport  Port=3  InitialOutput=0
  wires:
  Gain/1 -> c_2/1
  Sum2/1 -> Gain/1
  Math Function3/1 -> Sum2/4
  Math Function2/1 -> Sum2/3
  Math Function1/1 -> Sum2/2
  Math Function/1 -> Sum2/1
  y3/1 -> Math Function3/1, Sum1/2
  y2/1 -> Math Function2/1, Sum1/1
  x3/1 -> Math Function1/1, Sum/2
  x2/1 -> Math Function/1, Sum/1
  Sum1/1 -> beta_2/1
  Sum/1 -> alfa_2/1

== system HEMERO/Robots móviles/Control de robots móviles/Métodos basados en Teoría de Control/Seguimiento de caminos/Seguimiento de caminos (control lineal)/Cálculo de parámetros/Subsystem/Parametros de Curvatura/coordenada y c. curvatura/bloque_1 ==
  x1 : Inport  Port=1  PortWidth=-1  SampleTime=-1  DataType=auto
      settings: SignalType=auto
  x2 : Inport  Port=2  PortWidth=-1  SampleTime=-1  DataType=auto
      settings: SignalType=auto
  y1 : Inport  Port=3  PortWidth=-1  SampleTime=-1  DataType=auto
      settings: SignalType=auto
  y2 : Inport  Port=4  PortWidth=-1  SampleTime=-1  DataType=auto
      settings: SignalType=auto
  Gain : Gain  Gain=0.5  SaturateOnIntegerOverflow=on
  Math Function{,1..3} (4 alike) : Math  Operator=square  OutputSignalType=auto
  Sum : Sum  Inputs=-+  SaturateOnIntegerOverflow=on
  Sum1 : Sum  Inputs=-+  SaturateOnIntegerOverflow=on
  Sum2 : Sum  Inputs=-+-+  SaturateOnIntegerOverflow=on
  alfa_1 : Outport  Port=1  InitialOutput=0
  beta_1 : Outport  Port=2  InitialOutput=0
  c_1 : Outport  Port=3  InitialOutput=0
  wires:
  Gain/1 -> c_1/1
  Sum2/1 -> Gain/1
  Math Function3/1 -> Sum2/4
  Math Function2/1 -> Sum2/3
  Math Function1/1 -> Sum2/2
  Math Function/1 -> Sum2/1
  y2/1 -> Math Function3/1, Sum1/2
  y1/1 -> Math Function2/1, Sum1/1
  x2/1 -> Math Function1/1, Sum/2
  x1/1 -> Math Function/1, Sum/1
  Sum1/1 -> beta_1/1
  Sum/1 -> alfa_1/1

== system HEMERO/Robots móviles/Control de robots móviles/Métodos basados en Teoría de Control/Seguimiento de caminos/Seguimiento de caminos (control lineal)/Cálculo de parámetros/Subsystem/Parametros de Curvatura/coordenada y c. curvatura/bloque_2 ==
  x2 : Inport  Port=1  PortWidth=-1  SampleTime=-1  DataType=auto
      settings: SignalType=auto
  x3 : Inport  Port=2  PortWidth=-1  SampleTime=-1  DataType=auto
      settings: SignalType=auto
  y2 : Inport  Port=3  PortWidth=-1  SampleTime=-1  DataType=auto
      settings: SignalType=auto
  y3 : Inport  Port=4  PortWidth=-1  SampleTime=-1  DataType=auto
      settings: SignalType=auto
  Gain : Gain  Gain=0.5  SaturateOnIntegerOverflow=on
  Math Function{,1..3} (4 alike) : Math  Operator=square  OutputSignalType=auto
  Sum : Sum  Inputs=-+  SaturateOnIntegerOverflow=on
  Sum1 : Sum  Inputs=-+  SaturateOnIntegerOverflow=on
  Sum2 : Sum  Inputs=-+-+  SaturateOnIntegerOverflow=on
  alfa_2 : Outport  Port=1  InitialOutput=0
  beta_2 : Outport  Port=2  InitialOutput=0
  c_2 : Outport  Port=3  InitialOutput=0
  wires:
  Gain/1 -> c_2/1
  Sum2/1 -> Gain/1
  Math Function3/1 -> Sum2/4
  Math Function2/1 -> Sum2/3
  Math Function1/1 -> Sum2/2
  Math Function/1 -> Sum2/1
  y3/1 -> Math Function3/1, Sum1/2
  y2/1 -> Math Function2/1, Sum1/1
  x3/1 -> Math Function1/1, Sum/2
  x2/1 -> Math Function/1, Sum/1
  Sum1/1 -> beta_2/1
  Sum/1 -> alfa_2/1

== system HEMERO/Robots móviles/Control de robots móviles/Métodos basados en Teoría de Control/Seguimiento de caminos/Seguimiento de caminos (control no lineal)/Cálculo de parámetros/Subsystem/Parametros de Curvatura/coordenada x c. curvatura/bloque_1 ==
  x1 : Inport  Port=1  PortWidth=-1  SampleTime=-1  DataType=auto
      settings: SignalType=auto
  x2 : Inport  Port=2  PortWidth=-1  SampleTime=-1  DataType=auto
      settings: SignalType=auto
  y1 : Inport  Port=3  PortWidth=-1  SampleTime=-1  DataType=auto
      settings: SignalType=auto
  y2 : Inport  Port=4  PortWidth=-1  SampleTime=-1  DataType=auto
      settings: SignalType=auto
  Gain : Gain  Gain=0.5  SaturateOnIntegerOverflow=on
  Math Function{,1..3} (4 alike) : Math  Operator=square  OutputSignalType=auto
  Sum : Sum  Inputs=-+  SaturateOnIntegerOverflow=on
  Sum1 : Sum  Inputs=-+  SaturateOnIntegerOverflow=on
  Sum2 : Sum  Inputs=-+-+  SaturateOnIntegerOverflow=on
  alfa_1 : Outport  Port=1  InitialOutput=0
  beta_1 : Outport  Port=2  InitialOutput=0
  c_1 : Outport  Port=3  InitialOutput=0
  wires:
  Sum/1 -> alfa_1/1
  Sum1/1 -> beta_1/1
  x1/1 -> Sum/1, Math Function/1
  x2/1 -> Sum/2, Math Function1/1
  y1/1 -> Sum1/1, Math Function2/1
  y2/1 -> Sum1/2, Math Function3/1
  Math Function/1 -> Sum2/1
  Math Function1/1 -> Sum2/2
  Math Function2/1 -> Sum2/3
  Math Function3/1 -> Sum2/4
  Sum2/1 -> Gain/1
  Gain/1 -> c_1/1

== system HEMERO/Robots móviles/Control de robots móviles/Métodos basados en Teoría de Control/Seguimiento de caminos/Seguimiento de caminos (control no lineal)/Cálculo de parámetros/Subsystem/Parametros de Curvatura/coordenada x c. curvatura/bloque_2 ==
  x2 : Inport  Port=1  PortWidth=-1  SampleTime=-1  DataType=auto
      settings: SignalType=auto
  x3 : Inport  Port=2  PortWidth=-1  SampleTime=-1  DataType=auto
      settings: SignalType=auto
  y2 : Inport  Port=3  PortWidth=-1  SampleTime=-1  DataType=auto
      settings: SignalType=auto
  y3 : Inport  Port=4  PortWidth=-1  SampleTime=-1  DataType=auto
      settings: SignalType=auto
  Gain : Gain  Gain=0.5  SaturateOnIntegerOverflow=on
  Math Function{,1..3} (4 alike) : Math  Operator=square  OutputSignalType=auto
  Sum : Sum  Inputs=-+  SaturateOnIntegerOverflow=on
  Sum1 : Sum  Inputs=-+  SaturateOnIntegerOverflow=on
  Sum2 : Sum  Inputs=-+-+  SaturateOnIntegerOverflow=on
  alfa_2 : Outport  Port=1  InitialOutput=0
  beta_2 : Outport  Port=2  InitialOutput=0
  c_2 : Outport  Port=3  InitialOutput=0
  wires:
  Sum/1 -> alfa_2/1
  Sum1/1 -> beta_2/1
  x2/1 -> Sum/1, Math Function/1
  x3/1 -> Sum/2, Math Function1/1
  y2/1 -> Sum1/1, Math Function2/1
  y3/1 -> Sum1/2, Math Function3/1
  Math Function/1 -> Sum2/1
  Math Function1/1 -> Sum2/2
  Math Function2/1 -> Sum2/3
  Math Function3/1 -> Sum2/4
  Sum2/1 -> Gain/1
  Gain/1 -> c_2/1

== system HEMERO/Robots móviles/Control de robots móviles/Métodos basados en Teoría de Control/Seguimiento de caminos/Seguimiento de caminos (control no lineal)/Cálculo de parámetros/Subsystem/Parametros de Curvatura/coordenada y c. curvatura/bloque_1 ==
  x1 : Inport  Port=1  PortWidth=-1  SampleTime=-1  DataType=auto
      settings: SignalType=auto
  x2 : Inport  Port=2  PortWidth=-1  SampleTime=-1  DataType=auto
      settings: SignalType=auto
  y1 : Inport  Port=3  PortWidth=-1  SampleTime=-1  DataType=auto
      settings: SignalType=auto
  y2 : Inport  Port=4  PortWidth=-1  SampleTime=-1  DataType=auto
      settings: SignalType=auto
  Gain : Gain  Gain=0.5  SaturateOnIntegerOverflow=on
  Math Function{,1..3} (4 alike) : Math  Operator=square  OutputSignalType=auto
  Sum : Sum  Inputs=-+  SaturateOnIntegerOverflow=on
  Sum1 : Sum  Inputs=-+  SaturateOnIntegerOverflow=on
  Sum2 : Sum  Inputs=-+-+  SaturateOnIntegerOverflow=on
  alfa_1 : Outport  Port=1  InitialOutput=0
  beta_1 : Outport  Port=2  InitialOutput=0
  c_1 : Outport  Port=3  InitialOutput=0
  wires:
  Sum/1 -> alfa_1/1
  Sum1/1 -> beta_1/1
  x1/1 -> Sum/1, Math Function/1
  x2/1 -> Sum/2, Math Function1/1
  y1/1 -> Sum1/1, Math Function2/1
  y2/1 -> Sum1/2, Math Function3/1
  Math Function/1 -> Sum2/1
  Math Function1/1 -> Sum2/2
  Math Function2/1 -> Sum2/3
  Math Function3/1 -> Sum2/4
  Sum2/1 -> Gain/1
  Gain/1 -> c_1/1

== system HEMERO/Robots móviles/Control de robots móviles/Métodos basados en Teoría de Control/Seguimiento de caminos/Seguimiento de caminos (control no lineal)/Cálculo de parámetros/Subsystem/Parametros de Curvatura/coordenada y c. curvatura/bloque_2 ==
  x2 : Inport  Port=1  PortWidth=-1  SampleTime=-1  DataType=auto
      settings: SignalType=auto
  x3 : Inport  Port=2  PortWidth=-1  SampleTime=-1  DataType=auto
      settings: SignalType=auto
  y2 : Inport  Port=3  PortWidth=-1  SampleTime=-1  DataType=auto
      settings: SignalType=auto
  y3 : Inport  Port=4  PortWidth=-1  SampleTime=-1  DataType=auto
      settings: SignalType=auto
  Gain : Gain  Gain=0.5  SaturateOnIntegerOverflow=on
  Math Function{,1..3} (4 alike) : Math  Operator=square  OutputSignalType=auto
  Sum : Sum  Inputs=-+  SaturateOnIntegerOverflow=on
  Sum1 : Sum  Inputs=-+  SaturateOnIntegerOverflow=on
  Sum2 : Sum  Inputs=-+-+  SaturateOnIntegerOverflow=on
  alfa_2 : Outport  Port=1  InitialOutput=0
  beta_2 : Outport  Port=2  InitialOutput=0
  c_2 : Outport  Port=3  InitialOutput=0
  wires:
  Sum/1 -> alfa_2/1
  Sum1/1 -> beta_2/1
  x2/1 -> Sum/1, Math Function/1
  x3/1 -> Sum/2, Math Function1/1
  y2/1 -> Sum1/1, Math Function2/1
  y3/1 -> Sum1/2, Math Function3/1
  Math Function/1 -> Sum2/1
  Math Function1/1 -> Sum2/2
  Math Function2/1 -> Sum2/3
  Math Function3/1 -> Sum2/4
  Sum2/1 -> Gain/1
  Gain/1 -> c_2/1

== system HEMERO/Robots móviles/Control de robots móviles/Métodos basados en Teoría de Control/Seguimiento de trayectorias/Ejemplos/Ejemplo H.6.6/Seguimiento de trayectorias (Control lineal)/Cambio de variable/Cálculo de e3/Subsystem2 ==
  phi_gorro : Inport  Port=1  PortWidth=-1  SampleTime=-1  DataType=auto
      settings: SignalType=auto
  Constant1 : Constant  Value=360
  Constant2 : Constant  Value=360
  Sum1 : Sum  Inputs=-+  SaturateOnIntegerOverflow=on
  Sum2 : Sum  Inputs=++  SaturateOnIntegerOverflow=on
  Switch : Switch  Threshold=180
  Switch1 : Switch  Threshold=0
  Switch2 : Switch  Threshold=-180
  phi_go_mod : Outport  Port=1
  wires:
  Switch1/1 -> phi_go_mod/1
  Switch/1 -> Switch1/1
  Switch2/1 -> Switch1/3
  Constant1/1 -> Sum1/1
  Sum1/1 -> Switch/1
  Sum2/1 -> Switch2/3
  phi_gorro/1 -> Sum1/2, Switch1/2, Switch/3, Switch/2, Switch2/1, Switch2/2, Sum2/1
  Constant2/1 -> Sum2/2

== system HEMERO/Robots móviles/Control de robots móviles/Métodos basados en Teoría de Control/Seguimiento de trayectorias/Ejemplos/Ejemplo H.6.7/Seguimiento de trayectorias (Control lineal con escalado de velocidad)/Cambio de variable/Cálculo de e3/Subsystem2 ==
  phi_gorro : Inport  Port=1  PortWidth=-1  SampleTime=-1  DataType=auto
      settings: SignalType=auto
  Constant1 : Constant  Value=360
  Constant2 : Constant  Value=360
  Sum1 : Sum  Inputs=-+  SaturateOnIntegerOverflow=on
  Sum2 : Sum  Inputs=++  SaturateOnIntegerOverflow=on
  Switch : Switch  Threshold=180
  Switch1 : Switch  Threshold=0
  Switch2 : Switch  Threshold=-180
  phi_go_mod : Outport  Port=1
  wires:
  Switch1/1 -> phi_go_mod/1
  Switch/1 -> Switch1/1
  Switch2/1 -> Switch1/3
  Constant1/1 -> Sum1/1
  Sum1/1 -> Switch/1
  Sum2/1 -> Switch2/3
  phi_gorro/1 -> Sum1/2, Switch1/2, Switch/3, Switch/2, Switch2/1, Switch2/2, Sum2/1
  Constant2/1 -> Sum2/2

== system HEMERO/Robots móviles/Control de robots móviles/Métodos basados en Teoría de Control/Seguimiento de trayectorias/Ejemplos/Ejemplo H.6.8/Seguimiento de trayectorias (Control no lineal)/Cambio de variable/Cálculo de e3/Subsystem2 ==
  phi_gorro : Inport  Port=1  PortWidth=-1  SampleTime=-1  DataType=auto
      settings: SignalType=auto
  Constant1 : Constant  Value=360
  Constant2 : Constant  Value=360
  Sum1 : Sum  Inputs=-+  SaturateOnIntegerOverflow=on
  Sum2 : Sum  Inputs=++  SaturateOnIntegerOverflow=on
  Switch : Switch  Threshold=180
  Switch1 : Switch  Threshold=0
  Switch2 : Switch  Threshold=-180
  phi_go_mod : Outport  Port=1
  wires:
  Switch1/1 -> phi_go_mod/1
  Switch/1 -> Switch1/1
  Switch2/1 -> Switch1/3
  Constant1/1 -> Sum1/1
  Sum1/1 -> Switch/1
  Sum2/1 -> Switch2/3
  phi_gorro/1 -> Sum1/2, Switch1/2, Switch/3, Switch/2, Switch2/1, Switch2/2, Sum2/1
  Constant2/1 -> Sum2/2

== system HEMERO/Robots móviles/Control de robots móviles/Métodos basados en Teoría de Control/Seguimiento de caminos/Ejemplos/Ejemplo H.6.4/Seguimiento de caminos (control lineal)/Cálculo de parámetros/Subsystem/Parametros de Curvatura/Radio de  Curvatura ==
  x_g : Inport  Port=1  PortWidth=-1  SampleTime=-1  DataType=auto
      settings: SignalType=auto
  x_1 : Inport  Port=2  PortWidth=-1  SampleTime=-1  DataType=auto
      settings: SignalType=auto
  y_g : Inport  Port=3  PortWidth=-1  SampleTime=-1  DataType=auto
      settings: SignalType=auto
  y_1 : Inport  Port=4  PortWidth=-1  SampleTime=-1  DataType=auto
      settings: SignalType=auto
  Math Function : Math  Operator=square  OutputSignalType=auto
  Math Function1 : Math  Operator=sqrt  OutputSignalType=auto
  Math Function2 : Math  Operator=square  OutputSignalType=auto
  Sum : Sum  Inputs=+-  SaturateOnIntegerOverflow=on
  Sum1 : Sum  Inputs=+-  SaturateOnIntegerOverflow=on
  Sum2 : Sum  Inputs=++  SaturateOnIntegerOverflow=on
  R_c : Outport  Port=1  InitialOutput=0
  wires:
  Math Function1/1 -> R_c/1
  Sum2/1 -> Math Function1/1
  Math Function2/1 -> Sum2/2
  Math Function/1 -> Sum2/1
  Sum1/1 -> Math Function2/1
  Sum/1 -> Math Function/1
  y_g/1 -> Sum1/2
  y_1/1 -> Sum1/1
  x_1/1 -> Sum/1
  x_g/1 -> Sum/2
